simulink model "pwm_teste"  (R2015a)
settings: Solver=ode3  SolverMode=SingleTasking  StartTime=0.0  StopTime=Inf  FixedStep=0.0001  RelTol=1e-3
PostLoadFcn:
  | , if any(exist('dsrtsu_mdlpostloadfcn', 'file') == [2, 3, 6]), try dsrtsu_mdlpostloadfcn('Execute', bdroot); catch fprintf('Error in PostLoadFcn (dsrtsu_mdlpostloadfcn) for model "%s":\n %s\n', bdroot, lasterr); end, end,
libraries: rti2202miolib x6
settings Model: DSRTSU_INTERNAL_RTI_VER=450  DSRTSU_INTERNAL_RTI_TYPE=rti1006  DSRTSU_INTERNAL_RTIFPGA=40  CovMetricSettings=dwe  CovHtmlReporting=off  covSaveCumulativeToWorkspaceVar=off  CovSaveSingleToWorkspaceVar=off  CovExternalEMLEnable=on  Creator=Marcelo  LastModifiedBy=NSEE
settings SolverCC: ZeroCrossControl=DisableAll
settings DataIOCC: LimitDataPoints=off  SaveFormat=Dataset
settings OptimizationCC: BlockReduction=off  OptimizeBlockIOStorage=off  BufferReuse=off  GlobalBufferReuse=off  ExpressionFolding=off  LocalBlockOutputs=off
settings DebuggingCC: ParameterOverflowMsg=warning  SFUnexpectedBacktrackingDiag=error  SFNoUnconditionalDefaultTransitionDiag=error
settings HardwareCC: ProdBitPerPointer=64  ProdLargestAtomicFloat=Float  ProdIntDivRoundTo=Zero  ProdEndianess=LittleEndian  ProdHWDeviceType=Generic->Custom  TargetIntDivRoundTo=Zero  TargetEndianess=LittleEndian  TargetHWDeviceType=Generic->Custom
settings ModelReferenceCC: ModelReferenceMinAlgLoopOccurrences=on  PropagateSignalLabelsOutOfModel=on
settings RTWCC: SystemTargetFile=rti1006.tlc  MakeCommand=make_rti  TemplateMakefile=rti1006.tmf  Description=dSPACE DS1006 Hardware Platform
settings STFCustomTargetCC: GenerateSampleERTMain=off  ParMdlRefBuildCompliant=on  GeneratePreprocessorConditionals=Disable all  ERTCustomFileBanners=off  SupportNonInlinedSFcns=on  SupportVariableSizeSignals=off  MATLABClassNameForMDSCustomization=Simulink.SoftwareTarget.GRTCustomization  GRTInterface=on  SystemTargetFile=rti1006.tlc
settings GRTTargetCC: CompOptLevelCompliant=off  ConcurrentExecutionCompliant=off  CombineOutputUpdateFcns=off  MatFileLogging=off  CPPClassGenCompliant=off  GRTInterface=on  ExtModeMexFile=noextcomm

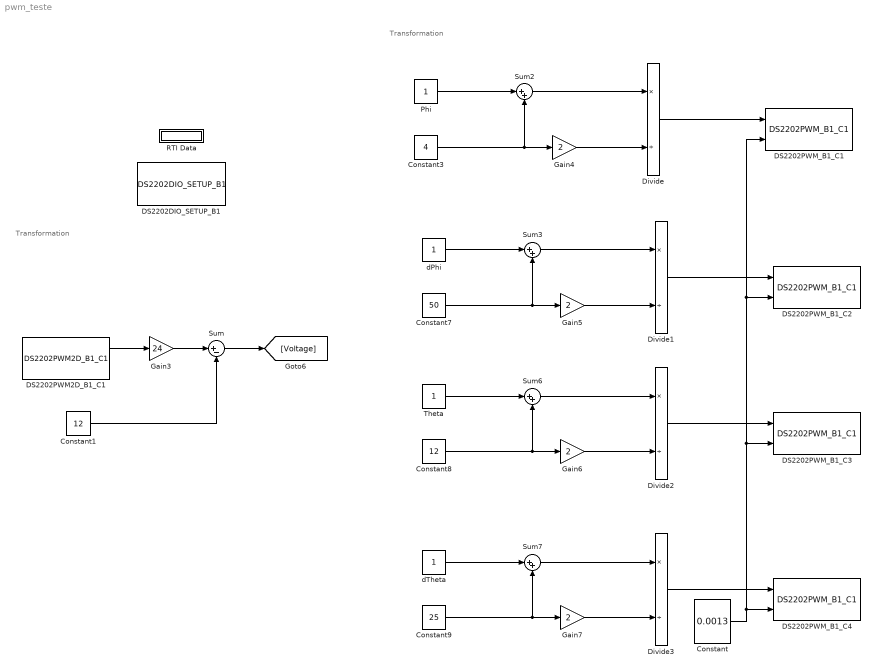
== system pwm_teste ==
  note: Transformation
  note: Transformation
  Constant : Constant  Value=0.0013
  Constant1 : Constant  Value=12
  Constant3 : Constant  Value=4
  Constant7 : Constant  Value=50
  Constant8 : Constant  Value=12
  Constant9 : Constant  Value=25
  DS2202DIO_SETUP_B1 : rti2202miolib/DS2202DIO_SETUP_B1  Reserved1=[]  Reserved2=[]  Reserved3=[]  Reserved4=[]  DSProperties=struct('RTI',struct('Version',uint32(2),'BlockType',struct('isSLSource',uint8(0),'isSLSink',uint8(0),'isHWSource',uint8(0),'isHWSink',uint8(0),'isSetup',uint8(1),'isInline',uint8(1),'isNonInline',uint8(0),'isInterrupt',uint8(0),'isChannelwise',uint8(0)),'IOBoardType',{{'DS2202','MIO'}},'UnitType','SETUP','Identifier','SETUP','DialogType','ML','BlockSet','NONE','SlaveProcessor','NONE'))  RTIBlockInterface=struct('OutputPortsWidth',int32(0),'OutputPortsActive',0,'BlockDisplay',{{['Digital I/O\n SETUP'],'center'}},'IconTransparency','on','InitLevel',2,'DialogFcn','gui2202diosetup','BlockName',struct('Token',{{'DS2202DIO_SETUP_B'}},'BlockParam',{{'BoardNo'}}),'MaskDescription',['Configures the threshold level and the termination mode for all digital IO'])  RTIBlockParameters=struct('BoardNo',{{1,'ON',[1 16]}},'TermMode',{{0,'OFF',[0 1]}},'BitInThresholdLevelCh1',{{'1.65','OFF',[1 23.8]}},'BitInThresholdLevelCh2',{{'1.65','OFF',[1 23.8]}},'BitInThresholdLevelCh3',{{'1.65','OFF',[1 23.8]}},'BitInThresholdLevelCh4',{{'1.65','OFF',[1 23.8]}},'BitInThresholdLevelCh5',{{'1.65','OFF',[1 23.8]}},'BitInThresholdLevelCh6',{{'1.65','OFF',[1 23.8]}},'BitInThresholdLevelCh7',{{'1.65','OFF',[1 23.8]}},'BitInThresholdLevelCh8',{{'1.65','OFF',[1 23.8]}},'BitInThresholdLevelCh9',{{'1.65','OFF',[1 23.8]}},'BitInThresholdLevelCh10',{{'1.65','OFF',[1 23.8]}},'BitInThresholdLevelCh11',{{'1.65','OFF',[1 23.8]}},'BitInThresholdLevelCh12',{{'1.65','OFF',[1 23.8]}},'BitInThresholdLevelCh13',{{'1.65','OFF',[1 23.8]}},'BitInThresholdLevelCh14',{{'1.65','OFF',[1 23.8]}},'BitInThresholdLevelCh15',{{'1.65','OFF',[1 23.8]}},'BitInThresholdLevelCh16',{{'1.65','OFF',[1 23.8]}},'BitInThresholdLevelCh17',{{'1.65','OFF',[1 23.8]}},'BitInThresholdLevelCh18',{{'1.65','OFF',[1 23.8]}},'BitInThresholdLevelCh19',{{'1.65','OFF',[1 23.8]}},'BitInThresholdLevelCh20',{{'1.65','OFF',[1 23.8]}},'BitInThresholdLevelCh21',{{'1.65','OFF',[1 23.8]}},'BitInThresholdLevelCh22',{{'1.65','OFF',[1 23.8]}},'BitInThresholdLevelCh23',{{'1.65','OFF',[1 23.8]}},'BitInThresholdLevelCh24',{{'1.65','OFF',[1 23.8]}},'BitInThresholdLevelCh25',{{'1.65','OFF',[1 23.8]}},'BitInThresholdLevelCh25_32',{{'1.65','OFF',[1 23.8]}},'BitInThresholdLevelCh33_38',{{'1.65','OFF',[1 23.8]}},'BitOutVBATRailsLOW',{{[1 1 1 1 1 1 1 1 1 1 1 1 1 1 1 1 1],'OFF',[]}},'BitOutVBATRailsVBAT1',{{[1 1 1 1 1 1 1 1 1 1 1 1 1 1 1 1 1],'OFF',[]}},'BitOutVBATRailsVBAT2',{{[0 0 0 0 0 0 0 0 0 0 0 0 0 0 0 0 0],'OFF',[]}},'PWMOutVBATRailsLOW',{{[1 1 1 1 1 1 1 1 1 1],'OFF',[]}},'PWMOutVBATRailsVBAT1',{{[1 1 1 1 1 1 1 1 1 1],'OFF',[]}},'PWMOutVBATRailsVBAT2',{{[0 0 0 0 0 0 0 0 0 0],'OFF',[]}},'TLCFileName',{{'rti2202setup','OFF',[]}})  RTISFcnParameters=struct('BoardNo','int32','TermMode','int32','BitInThresholdLevelCh1','double','BitInThresholdLevelCh2','double','BitInThresholdLevelCh3','double','BitInThresholdLevelCh4','double','BitInThresholdLevelCh5','double','BitInThresholdLevelCh6','double','BitInThresholdLevelCh7','double','BitInThresholdLevelCh8','double','BitInThresholdLevelCh9','double','BitInThresholdLevelCh10','double','BitInThresholdLevelCh11','double','BitInThresholdLevelCh12','double','BitInThresholdLevelCh13','double','BitInThresholdLevelCh14','double','BitInThresholdLevelCh15','double','BitInThresholdLevelCh16','double','BitInThresholdLevelCh17','double','BitInThresholdLevelCh18','double','BitInThresholdLevelCh19','double','BitInThresholdLevelCh20','double','BitInThresholdLevelCh21','double','BitInThresholdLevelCh22','double','BitInThresholdLevelCh23','double','BitInThresholdLevelCh24','double','BitInThresholdLevelCh25_32','double','BitInThresholdLevelCh33_38','double','BitOutVBATRailsLOW','int32','BitOutVBATRailsVBAT1','int32','BitOutVBATRailsVBAT2','int32','PWMOutVBATRailsLOW','int32','PWMOutVBATRailsVBAT1','int32','PWMOutVBATRailsVBAT2','int32','TLCFileName','char')  RTIBlockParaDefault=struct('BoardNo',1,'TermMode',0,'BitInThresholdLevelCh1',2.5,'BitInThresholdLevelCh2',2.5,'BitInThresholdLevelCh3',2.5,'BitInThresholdLevelCh4',2.5,'BitInThresholdLevelCh5',2.5,'BitInThresholdLevelCh6',2.5,'BitInThresholdLevelCh7',2.5,'BitInThresholdLevelCh8',2.5,'BitInThresholdLevelCh9',2.5,'BitInThresholdLevelCh10',2.5,'BitInThresholdLevelCh11',2.5,'BitInThresholdLevelCh12',2.5,'BitInThresholdLevelCh13',2.5,'BitInThresholdLevelCh14',2.5,'BitInThresholdLevelCh15',2.5,'BitInThresholdLevelCh16',2.5,'BitInThresholdLevelCh17',2.5,'BitInThresholdLevelCh18',2.5,'BitInThresholdLevelCh19',2.5,'BitInThresholdLevelCh20',2.5,'BitInThresholdLevelCh21',2.5,'BitInThresholdLevelCh22',2.5,'BitInThresholdLevelCh23',2.5,'BitInThresholdLevelCh24',2.5,'BitInThresholdLevelCh25',2.5,'BitInThresholdLevelCh25_32',2.5,'BitInThresholdLevelCh33_38',2.5,'BitOutVBATRailsLOW',[1 1 1 1 1 1 1 1 1 1 1 1 1 1 1 1 1],'BitOutVBATRailsVBAT1',[1 1 1 1 1 1 1 1 1 1 1 1 1 1 1 1 1],'BitOutVBATRailsVBAT2',[0 0 0 0 0 0 0 0 0 0 0 0 0 0 0 0 0],'PWMOutVBATRailsLOW',[1 1 1 1 1 1 1 1 1 1],'PWMOutVBATRailsVBAT1',[1 1 1 1 1 1 1 1 1 1],'PWMOutVBATRailsVBAT2',[0 0 0 0 0 0 0 0 0 0],'TLCFileName','rti2202setup')
  DS2202PWM2D_B1_C1 : rti2202miolib/DS2202PWM2D_B1_C1  Reserved1=[]  Reserved2=[]  Reserved3=[]  Reserved4=[]  DSProperties=struct('RTI',struct('Version',uint32(1),'BlockType',struct('isSLSource',uint8(1),'isSLSink',uint8(0),'isHWSource',uint8(1),'isHWSink',uint8(0),'isSetup',uint8(0),'isInline',uint8(1),'isNonInline',uint8(0),'isInterrupt',uint8(0),'isChannelwise',uint8(1)),'IOBoardType',{{'DS2202','MIO'}},'UnitType','PWM','Identifier','PWM2D','DialogType','ML','BlockSet','NONE','SlaveProcessor','NONE'))  RTIBlockInterface=struct('OutputPortsWidth',int32([1 1]),'OutputPortsActive',[1 1],'OutputPortsName',{{['Duty Cycle'],'Period'}},'IconTransparency','on','InitLevel',2,'DialogFcn','gui2202pwm2d','BlockName',struct('Token',{{'DS2202PWM2D_B','_C'}},'BlockParam',{{'BoardNo','ChannelNo'}}),'MaskDescription',['Provides read access to the pulse width of square-wave-type signals.'])  RTIBlockParameters=struct('BoardNo',{{1,'ON',[1 16]}},'ChannelNo',{{1,'ON',[1 24]}},'UpdateMode',{{1,'ON',[1 2]}},'PeriodRange',{{7,'OFF',[1 16]}},'TLCFileName',{{'rti2202pwm2d','OFF',[]}})  RTISFcnParameters=struct('BoardNo','int32','ChannelNo','int32','UpdateMode','int32','PeriodRange','int32','TLCFileName','char')  RTIBlockParaDefault=struct('BoardNo',1,'ChannelNo',1,'UpdateMode',1,'PeriodRange',7,'TLCFileName','rti2202pwm2d')
  DS2202PWM_B1_C1 : rti2202miolib/DS2202PWM_B1_C1  Reserved1=[]  Reserved2=[]  Reserved3=[]  Reserved4=[]  DSProperties=struct('RTI',struct('Version',uint32(1),'BlockType',struct('isSLSource',uint8(0),'isSLSink',uint8(1),'isHWSource',uint8(0),'isHWSink',uint8(1),'isSetup',uint8(0),'isInline',uint8(1),'isNonInline',uint8(0),'isInterrupt',uint8(0),'isChannelwise',uint8(1)),'IOBoardType',{{'DS2202','MIO'}},'UnitType','PWM','Identifier','PWM','DialogType','ML','BlockSet','NONE','SlaveProcessor','NONE'))  RTIBlockInterface=struct('InputPortsWidth',int32([1 1]),'InputPortsActive',[1 1],'InputPortsName',{{['Duty Cycle'],'Period'}},'IconTransparency','on','InitLevel',2,'DialogFcn','gui2202pwm','BlockName',struct('Token',{{'DS2202PWM_B','_C'}},'BlockParam',{{'BoardNo','ChannelNo'}}),'MaskDescription',['Generation of a square-wave-type signal for a given period and duty cycle.'])  RTIBlockParameters=struct('BoardNo',{{1,'ON',[1 16]}},'ChannelNo',{{1,'ON',[1 9]}},'UpdateMode',{{1,'ON',[1 2]}},'PeriodRange',{{4,'OFF',[1 16]}},'DutyCycleInitValue',{{'0','OFF',[0 1]}},'PeriodInitValue',{{'5e-05','OFF',[]}},'DutyCyclePeriodTermMode',{{0,'OFF',[0 1]}},'DutyCycleTermValue',{{'0','OFF',[0 1]}},'PeriodTermValue',{{'5e-05','OFF',[]}},'TLCFileName',{{'rti2202pwm','OFF',[]}})  RTISFcnParameters=struct('BoardNo','int32','ChannelNo','int32','UpdateMode','int32','PeriodRange','int32','DutyCycleInitValue','double','PeriodInitValue','double','DutyCyclePeriodTermMode','int32','DutyCycleTermValue','double','PeriodTermValue','double','TLCFileName','char')  RTIBlockParaDefault=struct('BoardNo',1,'ChannelNo',1,'UpdateMode',1,'PeriodRange',7,'DutyCycleInitValue',0,'PeriodInitValue',5e-05,'DutyCyclePeriodTermMode',0,'DutyCycleTermValue',0,'PeriodTermValue',5e-05,'TLCFileName','rti2202pwm')
  DS2202PWM_B1_C2 : rti2202miolib/DS2202PWM_B1_C1  Reserved1=[]  Reserved2=[]  Reserved3=[]  Reserved4=[]  DSProperties=struct('RTI',struct('Version',uint32(1),'BlockType',struct('isSLSource',uint8(0),'isSLSink',uint8(1),'isHWSource',uint8(0),'isHWSink',uint8(1),'isSetup',uint8(0),'isInline',uint8(1),'isNonInline',uint8(0),'isInterrupt',uint8(0),'isChannelwise',uint8(1)),'IOBoardType',{{'DS2202','MIO'}},'UnitType','PWM','Identifier','PWM','DialogType','ML','BlockSet','NONE','SlaveProcessor','NONE'))  RTIBlockInterface=struct('InputPortsWidth',int32([1 1]),'InputPortsActive',[1 1],'InputPortsName',{{['Duty Cycle'],'Period'}},'IconTransparency','on','InitLevel',2,'DialogFcn','gui2202pwm','BlockName',struct('Token',{{'DS2202PWM_B','_C'}},'BlockParam',{{'BoardNo','ChannelNo'}}),'MaskDescription',['Generation of a square-wave-type signal for a given period and duty cycle.'])  RTIBlockParameters=struct('BoardNo',{{1,'ON',[1 16]}},'ChannelNo',{{2,'ON',[1 9]}},'UpdateMode',{{1,'ON',[1 2]}},'PeriodRange',{{4,'OFF',[1 16]}},'DutyCycleInitValue',{{'0','OFF',[0 1]}},'PeriodInitValue',{{'5e-05','OFF',[]}},'DutyCyclePeriodTermMode',{{0,'OFF',[0 1]}},'DutyCycleTermValue',{{'0','OFF',[0 1]}},'PeriodTermValue',{{'5e-05','OFF',[]}},'TLCFileName',{{'rti2202pwm','OFF',[]}})  RTISFcnParameters=struct('BoardNo','int32','ChannelNo','int32','UpdateMode','int32','PeriodRange','int32','DutyCycleInitValue','double','PeriodInitValue','double','DutyCyclePeriodTermMode','int32','DutyCycleTermValue','double','PeriodTermValue','double','TLCFileName','char')  RTIBlockParaDefault=struct('BoardNo',1,'ChannelNo',1,'UpdateMode',1,'PeriodRange',7,'DutyCycleInitValue',0,'PeriodInitValue',5e-05,'DutyCyclePeriodTermMode',0,'DutyCycleTermValue',0,'PeriodTermValue',5e-05,'TLCFileName','rti2202pwm')
  DS2202PWM_B1_C3 : rti2202miolib/DS2202PWM_B1_C1  Reserved1=[]  Reserved2=[]  Reserved3=[]  Reserved4=[]  DSProperties=struct('RTI',struct('Version',uint32(1),'BlockType',struct('isSLSource',uint8(0),'isSLSink',uint8(1),'isHWSource',uint8(0),'isHWSink',uint8(1),'isSetup',uint8(0),'isInline',uint8(1),'isNonInline',uint8(0),'isInterrupt',uint8(0),'isChannelwise',uint8(1)),'IOBoardType',{{'DS2202','MIO'}},'UnitType','PWM','Identifier','PWM','DialogType','ML','BlockSet','NONE','SlaveProcessor','NONE'))  RTIBlockInterface=struct('InputPortsWidth',int32([1 1]),'InputPortsActive',[1 1],'InputPortsName',{{['Duty Cycle'],'Period'}},'IconTransparency','on','InitLevel',2,'DialogFcn','gui2202pwm','BlockName',struct('Token',{{'DS2202PWM_B','_C'}},'BlockParam',{{'BoardNo','ChannelNo'}}),'MaskDescription',['Generation of a square-wave-type signal for a given period and duty cycle.'])  RTIBlockParameters=struct('BoardNo',{{1,'ON',[1 16]}},'ChannelNo',{{3,'ON',[1 9]}},'UpdateMode',{{1,'ON',[1 2]}},'PeriodRange',{{4,'OFF',[1 16]}},'DutyCycleInitValue',{{'0','OFF',[0 1]}},'PeriodInitValue',{{'5e-05','OFF',[]}},'DutyCyclePeriodTermMode',{{0,'OFF',[0 1]}},'DutyCycleTermValue',{{'0','OFF',[0 1]}},'PeriodTermValue',{{'5e-05','OFF',[]}},'TLCFileName',{{'rti2202pwm','OFF',[]}})  RTISFcnParameters=struct('BoardNo','int32','ChannelNo','int32','UpdateMode','int32','PeriodRange','int32','DutyCycleInitValue','double','PeriodInitValue','double','DutyCyclePeriodTermMode','int32','DutyCycleTermValue','double','PeriodTermValue','double','TLCFileName','char')  RTIBlockParaDefault=struct('BoardNo',1,'ChannelNo',1,'UpdateMode',1,'PeriodRange',7,'DutyCycleInitValue',0,'PeriodInitValue',5e-05,'DutyCyclePeriodTermMode',0,'DutyCycleTermValue',0,'PeriodTermValue',5e-05,'TLCFileName','rti2202pwm')
  DS2202PWM_B1_C4 : rti2202miolib/DS2202PWM_B1_C1  Reserved1=[]  Reserved2=[]  Reserved3=[]  Reserved4=[]  DSProperties=struct('RTI',struct('Version',uint32(1),'BlockType',struct('isSLSource',uint8(0),'isSLSink',uint8(1),'isHWSource',uint8(0),'isHWSink',uint8(1),'isSetup',uint8(0),'isInline',uint8(1),'isNonInline',uint8(0),'isInterrupt',uint8(0),'isChannelwise',uint8(1)),'IOBoardType',{{'DS2202','MIO'}},'UnitType','PWM','Identifier','PWM','DialogType','ML','BlockSet','NONE','SlaveProcessor','NONE'))  RTIBlockInterface=struct('InputPortsWidth',int32([1 1]),'InputPortsActive',[1 1],'InputPortsName',{{['Duty Cycle'],'Period'}},'IconTransparency','on','InitLevel',2,'DialogFcn','gui2202pwm','BlockName',struct('Token',{{'DS2202PWM_B','_C'}},'BlockParam',{{'BoardNo','ChannelNo'}}),'MaskDescription',['Generation of a square-wave-type signal for a given period and duty cycle.'])  RTIBlockParameters=struct('BoardNo',{{1,'ON',[1 16]}},'ChannelNo',{{4,'ON',[1 9]}},'UpdateMode',{{1,'ON',[1 2]}},'PeriodRange',{{4,'OFF',[1 16]}},'DutyCycleInitValue',{{'0','OFF',[0 1]}},'PeriodInitValue',{{'5e-05','OFF',[]}},'DutyCyclePeriodTermMode',{{0,'OFF',[0 1]}},'DutyCycleTermValue',{{'0','OFF',[0 1]}},'PeriodTermValue',{{'5e-05','OFF',[]}},'TLCFileName',{{'rti2202pwm','OFF',[]}})  RTISFcnParameters=struct('BoardNo','int32','ChannelNo','int32','UpdateMode','int32','PeriodRange','int32','DutyCycleInitValue','double','PeriodInitValue','double','DutyCyclePeriodTermMode','int32','DutyCycleTermValue','double','PeriodTermValue','double','TLCFileName','char')  RTIBlockParaDefault=struct('BoardNo',1,'ChannelNo',1,'UpdateMode',1,'PeriodRange',7,'DutyCycleInitValue',0,'PeriodInitValue',5e-05,'DutyCyclePeriodTermMode',0,'DutyCycleTermValue',0,'PeriodTermValue',5e-05,'TLCFileName','rti2202pwm')
  Divide{,1..3} (4 alike) : Product  Inputs=*/
  Gain3 : Gain  Gain=24
  Gain{4..7} (4 alike) : Gain  Gain=2
  Phi : Constant
  RTI Data : Subsystem  Tag=struct('RTIDataServer',struct('RTIDataServerVs','2','RTIModelDescription','struct(''main'',''pwm_teste'',''sub'','''',''isMp'',0)'))  LoadFcn="if exist('rtidc'), try,  rtidc('DataHostBlockClbLoad', gcbh); catch, disp(['Warning: ''LoadFcn'' for RTI Data block failed: ' lasterr]); end, end,"  mask(RTI_DATA_HOST){}
      mask help:
      | RTI Data Block.
      | This block is used by RTI to store internal model-dependent data.
      | Please keep this block on the root level of the model. Deleting this block will result in data loss.
      |
      | NEVER DELETE OR COPY THIS BLOCK!
      settings: CopyFcn="if exist('rtidc'), try,  rtidc('DataHostBlockClbCopy', gcbh); catch, disp(['Warning: ''CopyFcn'' for RTI Data block failed: ' lasterr]); end, end,"  DeleteFcn="if exist('rtidc'), try,  rtidc('DataHostBlockClbDelete', gcbh); catch, disp(['Warning: ''DeleteFcn'' for RTI Data block failed: ' lasterr]); end, end,"  ModelCloseFcn="if exist('rtidc'), try,  rtidc('DataHostBlockClbModelClose', gcbh); catch, disp(['Warning: ''ModelCloseFcn'' for RTI Data block failed: ' lasterr]); end, end,"  PreSaveFcn="if exist('rtidc'), try,  rtidc('DataHostBlockClbPreSave', gcbh); catch, disp(['Warning: ''PreSaveFcn'' for RTI Data block failed: ' lasterr]); end, end,"  PostSaveFcn="if exist('rtidc'), try,  rtidc('DataHostBlockClbPostSave', gcbh); catch, disp(['Warning: ''PostSaveFcn'' for RTI Data block failed: ' lasterr]); end, end,"  NameChangeFcn="if exist('rtidc'), try,  rtidc('DataHostBlockClbNameChange', gcbh); catch, disp(['Warning: ''NameChangeFcn'' for RTI Data block failed: ' lasterr]); end, end,"
      mask Help:
      | RTI Data Block.
      | This block is used by RTI to store internal model-dependent data.
      | Please keep this block on the root level of the model. Deleting this block will result in data loss.
      | 
      | NEVER DELETE OR COPY THIS BLOCK!
      mask Display:
      | text(0.5, 0.5, 'RTI Data', 'HorizontalAlignment', 'center');
      | plot([1 0]);
  Sum : Sum  Inputs=|+-
  Sum{2..3,6..7} (4 alike) : Sum  Inputs=|++
  Theta : Constant
  dPhi : Constant
  dTheta : Constant
  wires:
  DS2202PWM2D_B1_C1/1 -> Gain3/1
  Gain3/1 -> Sum/1
  Constant1/1 -> Sum/2
  Sum/1 -> [Voltage]
  Phi/1 -> Sum2/1
  Sum2/1 -> Divide/1
  Constant3/1 -> Gain4/1, Sum2/2
  Gain4/1 -> Divide/2
  Divide/1 -> DS2202PWM_B1_C1/1
  dPhi/1 -> Sum3/1
  Sum3/1 -> Divide1/1
  Constant7/1 -> Gain5/1, Sum3/2
  Gain5/1 -> Divide1/2
  Divide1/1 -> DS2202PWM_B1_C2/1
  Theta/1 -> Sum6/1
  Sum6/1 -> Divide2/1
  Constant8/1 -> Gain6/1, Sum6/2
  Gain6/1 -> Divide2/2
  Divide2/1 -> DS2202PWM_B1_C3/1
  dTheta/1 -> Sum7/1
  Sum7/1 -> Divide3/1
  Constant9/1 -> Gain7/1, Sum7/2
  Gain7/1 -> Divide3/2
  Divide3/1 -> DS2202PWM_B1_C4/1
  Constant/1 -> DS2202PWM_B1_C1/2, DS2202PWM_B1_C2/2, DS2202PWM_B1_C3/2, DS2202PWM_B1_C4/2

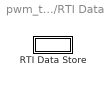
== system pwm_teste/RTI Data ==
  RTI Data Store : Subsystem  Tag="struct('private',struct('version',struct('dsVer',uint32(2),'dsVerCreation',uint32(2),'RTI',struct('ver','7.3','type','RTI1006')),'access',struct('type','Model','isPerm',1,'created',['02-Oct-2018 16:40:55'],'modified',['26-Oct-2018 21:59:42'],'location','')),'public',struct('main',struct('data',[]),'sub',struct('name',{{'pwm_teste'}},'data',{{struct('TH',struct('thTaskInfo',struct('taskType',{'TIMER','HWINT','TMRINT','SWINT','GLINT'},'tasksNumOf',{1,0,0,0,0},'srcIds',{{'TIMERA'},{},{},{},{}},'taskNames',{{['Timer Task 1']},{},{},{},{}})),'th_tc',struct('dataType','TASK','taskGroupId','','taskGroupList',{{}},'taskSchedulingPolicy','FCFS','taskType','TIMER','blkh',-1,'srcId','TIMERA','srcSgnName',['Timer A interrupt'],'srcCpuName','','taskName',['Timer Task 1  [0.0001] s'],'taskNameDisplayExt','','smplTime',0.0001,'smplTimeOffs',0,'hasFixedPriority',0,'priority',1,'hasFixedOvc',0,'ovcType',1,'ovcMax',1),'tc_th',struct('dataType','TASK','taskGroupId','','taskGroupList',{{}},'taskSchedulingPolicy','FCFS','taskType','TIMER','blkh',-1,'srcId','TIMERA','srcSgnName',['Timer A interrupt'],'srcCpuName','','taskName',['Timer Task 1  [0.0001] s'],'taskNameDisplayExt','','smplTime',0.0001,'smplTimeOffs',0,'hasFixedPriority',0,'priority',1,'hasFixedOvc',0,'ovcType',1,'ovcMax',1))}})))"  mask(RTI_DATA_STORE){}
      mask help:
      | RTI Data Store Block. This block is used by RTI to store internal model dependent data. Deleting this block will result in data loss.
      |
      | NEVER DELETE, COPY, OR MODIFY THIS BLOCK!
      mask Help:
      | RTI Data Store Block. This block is used by RTI to store internal model dependent data. Deleting this block will result in data loss.
      | 
      | NEVER DELETE, COPY, OR MODIFY THIS BLOCK!
      mask Display: text(0.5, 0.5, ' ', 'HorizontalAlignment', 'center');

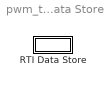
== system pwm_teste/RTI Data/RTI Data Store ==
  RTI Data Store : Subsystem  mask(RTI_DATA_STORE){}
      mask help:
      | RTI Data Store Block. This block is used by RTI to store internal model dependent data. Deleting this block will result in data loss.
      |
      | NEVER DELETE, COPY, OR MODIFY THIS BLOCK!
      mask Help:
      | RTI Data Store Block. This block is used by RTI to store internal model dependent data. Deleting this block will result in data loss.
      | 
      | NEVER DELETE, COPY, OR MODIFY THIS BLOCK!
      mask Display: text(0.5, 0.5, ' ', 'HorizontalAlignment', 'center');

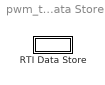
== system pwm_teste/RTI Data/RTI Data Store/RTI Data Store ==
  RTI Data Store : Subsystem  mask(RTI_DATA_STORE){}
      mask help:
      | RTI Data Store Block. This block is used by RTI to store internal model dependent data. Deleting this block will result in data loss.
      |
      | NEVER DELETE, COPY, OR MODIFY THIS BLOCK!
      mask Help:
      | RTI Data Store Block. This block is used by RTI to store internal model dependent data. Deleting this block will result in data loss.
      | 
      | NEVER DELETE, COPY, OR MODIFY THIS BLOCK!
      mask Display: text(0.5, 0.5, ' ', 'HorizontalAlignment', 'center');

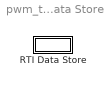
== system pwm_teste/RTI Data/RTI Data Store/RTI Data Store/RTI Data Store ==
  RTI Data Store : Subsystem  mask(RTI_DATA_STORE){}
      mask help:
      | RTI Data Store Block. This block is used by RTI to store internal model dependent data. Deleting this block will result in data loss.
      |
      | NEVER DELETE, COPY, OR MODIFY THIS BLOCK!
      mask Help:
      | RTI Data Store Block. This block is used by RTI to store internal model dependent data. Deleting this block will result in data loss.
      | 
      | NEVER DELETE, COPY, OR MODIFY THIS BLOCK!
      mask Display: text(0.5, 0.5, ' ', 'HorizontalAlignment', 'center');

== system pwm_teste/RTI Data/RTI Data Store/RTI Data Store/RTI Data Store/RTI Data Store ==
